simulink model "ME19B031_PROJECT_2"  (R2021a)
settings: Solver=VariableStepAuto  StartTime=0.0  StopTime=10.0  RelTol=1e-3
libraries: simulink_extras x7, pid_lib x2
settings Model: Creator=nayin  LastModifiedBy=nayin
settings SolverCC: ZeroCrossAlgorithm=Adaptive
settings DebuggingCC: IgnoredZcDiagnostic=none

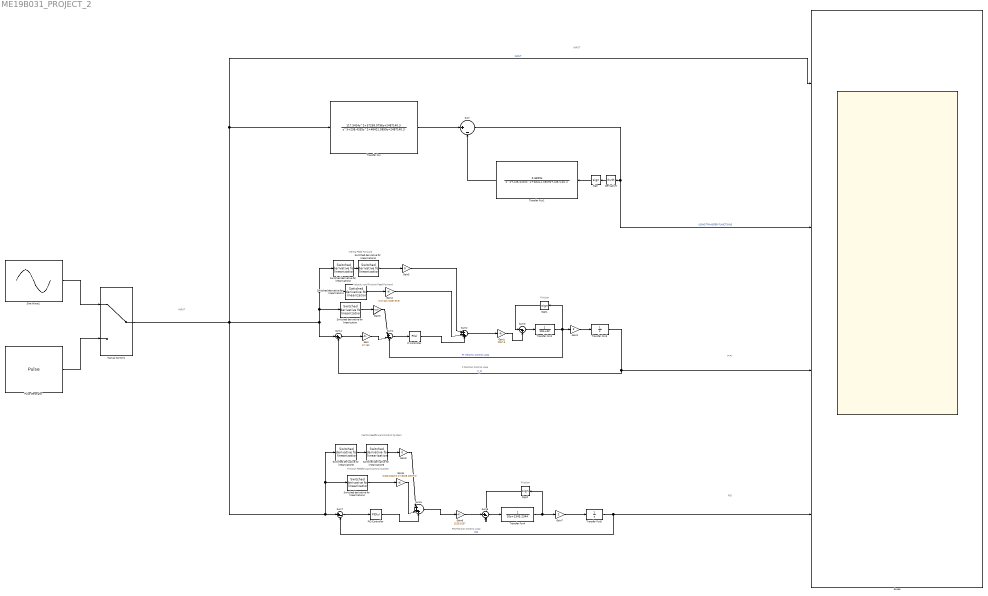
== system ME19B031_PROJECT_2 ==
  note: INPUT
  note: INPUT
  note: PID
  note: P-PI
  note: Velocity and Friction Feed Forward
  note: Inertia Feed Forward
  note: Friction
  note: P Position Control Loop
  note: PID Position Control Loop
  note: Inertia Feedforward Control System
  note: Friction Feedforward Control System
  note: Friction
  Derivative : Derivative
  Gain : Gain  Gain=37.133
  Gain1 : Gain  Gain=2057.6
  Gain2 : Gain  Gain=3
  Gain3 : Gain  Gain=0.5/3
  Gain4 : Gain  Gain=(0.1*42)/(2057.6*3)
  Gain5 : Gain  Gain=0
  Gain6 : Gain  Gain=3228.1057
  Gain7 : Gain  Gain=3
  Gain8 : Gain  Gain=(1343.2344*0.1)/(3228.1057*3)
  Gain9 : Gain  Gain=0
  Manual Switch1 : ManualSwitch
  PI Controller : pid_lib/PID Controller  Controller=PI  Form=Parallel  TimeDomain=Continuous-time  UseExternalTs=off  SampleTime=-1  IntegratorMethod=Forward Euler  FilterMethod=Forward Euler  ControllerParametersSource=internal  P=1.13838  I=108.5  D=0  UseFilter=on  N=100  TunerSelectOption=Transfer Function Based (PID Tuner App)  InitialConditionSource=internal  InitialConditionForIntegrator=0  InitialConditionForFilter=0  DifferentiatorICPrevScaledInput=0  ExternalReset=none  TrackingMode=off  Kt=1  LimitOutput=off  SatLimitsSource=internal  UpperSaturationLimit=inf  LowerSaturationLimit=-inf  LinearizeAsGain=on  AntiWindupMode=none  Kb=1  POutMin=[]  POutMax=[]  IOutMin=[]  IOutMax=[]  DOutMin=[]  DOutMax=[]  NOutMin=[]  NOutMax=[]  SumOutMin=[]  SumOutMax=[]  SaturationOutMin=[]  SaturationOutMax=[]  PParamMin=[]  PParamMax=[]  IParamMin=[]  IParamMax=[]  DParamMin=[]  DParamMax=[]  NParamMin=[]  NParamMax=[]  KbParamMin=[]  KbParamMax=[]  KtParamMin=[]  KtParamMax=[]  KbOutMin=[]  KbOutMax=[]  KtOutMin=[]  KtOutMax=[]  IntegratorOutMin=[]  IntegratorOutMax=[]  FilterOutMin=[]  FilterOutMax=[]  SumI1OutMin=[]  SumI1OutMax=[]  SumI2OutMin=[]  SumI2OutMax=[]  SumI3OutMin=[]  SumI3OutMax=[]  SumI4OutMin=[]  SumI4OutMax=[]  SumDOutMin=[]  SumDOutMax=[]  DifferentiatorOutMin=[]  DifferentiatorOutMax=[]  FilterDiffOutCoefMin=[]  FilterDiffOutCoefMax=[]  ReciprocalOutMin=[]  ReciprocalOutMax=[]  SumDenOutMin=[]  SumDenOutMax=[]  SumNumOutMin=[]  SumNumOutMax=[]  DivideOutMin=[]  DivideOutMax=[]  UdiffTsProdOutMin=[]  UdiffTsProdOutMax=[]  NTsProdOutMin=[]  NTsProdOutMax=[]  UintegralTsProdOutMin=[]  UintegralTsProdOutMax=[]  UngainTsProdOutMin=[]  UngainTsProdOutMax=[]  IntegratorContinuousStateAttributes=''  IntegratorStateMustResolveToSignalObject=off  IntegratorRTWStateStorageClass=Auto  FilterContinuousStateAttributes=''  FilterStateMustResolveToSignalObject=off  FilterRTWStateStorageClass=Auto  ParallelPVariant=InternalParameters  IdealPVariant=Disabled  IVariant=InternalParameters  DVariant=Disabled  IntegratorVariant=Continuous  SatVariant=Disabled  AWVariant=Passthrough  PCopyVariant=Disabled  TRVariant=Disabled  FdbkBlocksVariant=Forward  IdealPFdbkVariant=Disabled  SatFdbkVariant=Disabled  DerivativeFilterVariant=Disabled  NVariant=Disabled  NCopyVariant=Disabled_SignalSpec  FilterICVariant=Disabled  IntegratorICVariant=InternalICs  ExternalResetVariant=Disabled  TRSumVariant=Passthrough  SumFdbkVariant=Disabled  SumVariant=Sum_PI  TsampFilterVariant=InternalTs  TsampNgainVariant=Passthrough  TsampIntegralVariant=Passthrough  ExternalSaturationOutDataTypeStr=Inherit: Same as second input
  PID Controller : pid_lib/PID Controller  Controller=PID  Form=Parallel  TimeDomain=Continuous-time  UseExternalTs=off  SampleTime=-1  IntegratorMethod=Forward Euler  FilterMethod=Forward Euler  ControllerParametersSource=internal  P=50  I=2568.2141  D=2.323356  UseFilter=on  N=100  TunerSelectOption=Transfer Function Based (PID Tuner App)  InitialConditionSource=internal  InitialConditionForIntegrator=0  InitialConditionForFilter=0  DifferentiatorICPrevScaledInput=0  ExternalReset=none  TrackingMode=off  Kt=1  LimitOutput=off  SatLimitsSource=internal  UpperSaturationLimit=inf  LowerSaturationLimit=-inf  LinearizeAsGain=on  AntiWindupMode=none  Kb=1  POutMin=[]  POutMax=[]  IOutMin=[]  IOutMax=[]  DOutMin=[]  DOutMax=[]  NOutMin=[]  NOutMax=[]  SumOutMin=[]  SumOutMax=[]  SaturationOutMin=[]  SaturationOutMax=[]  PParamMin=[]  PParamMax=[]  IParamMin=[]  IParamMax=[]  DParamMin=[]  DParamMax=[]  NParamMin=[]  NParamMax=[]  KbParamMin=[]  KbParamMax=[]  KtParamMin=[]  KtParamMax=[]  KbOutMin=[]  KbOutMax=[]  KtOutMin=[]  KtOutMax=[]  IntegratorOutMin=[]  IntegratorOutMax=[]  FilterOutMin=[]  FilterOutMax=[]  SumI1OutMin=[]  SumI1OutMax=[]  SumI2OutMin=[]  SumI2OutMax=[]  SumI3OutMin=[]  SumI3OutMax=[]  SumI4OutMin=[]  SumI4OutMax=[]  SumDOutMin=[]  SumDOutMax=[]  DifferentiatorOutMin=[]  DifferentiatorOutMax=[]  FilterDiffOutCoefMin=[]  FilterDiffOutCoefMax=[]  ReciprocalOutMin=[]  ReciprocalOutMax=[]  SumDenOutMin=[]  SumDenOutMax=[]  SumNumOutMin=[]  SumNumOutMax=[]  DivideOutMin=[]  DivideOutMax=[]  UdiffTsProdOutMin=[]  UdiffTsProdOutMax=[]  NTsProdOutMin=[]  NTsProdOutMax=[]  UintegralTsProdOutMin=[]  UintegralTsProdOutMax=[]  UngainTsProdOutMin=[]  UngainTsProdOutMax=[]  IntegratorContinuousStateAttributes=''  IntegratorStateMustResolveToSignalObject=off  IntegratorRTWStateStorageClass=Auto  FilterContinuousStateAttributes=''  FilterStateMustResolveToSignalObject=off  FilterRTWStateStorageClass=Auto  ParallelPVariant=InternalParameters  IdealPVariant=Disabled  IVariant=InternalParameters  DVariant=InternalParameters  IntegratorVariant=Continuous  SatVariant=Disabled  AWVariant=Passthrough  PCopyVariant=Disabled  TRVariant=Disabled  FdbkBlocksVariant=Forward  IdealPFdbkVariant=Disabled  SatFdbkVariant=Disabled  DerivativeFilterVariant=ContFilter  NVariant=InternalParameters  NCopyVariant=Disabled  FilterICVariant=InternalICsFilter  IntegratorICVariant=InternalICs  ExternalResetVariant=Disabled  TRSumVariant=Passthrough  SumFdbkVariant=Disabled  SumVariant=Sum_PID  TsampFilterVariant=InternalTs  TsampNgainVariant=Passthrough  TsampIntegralVariant=Passthrough  ExternalSaturationOutDataTypeStr=Inherit: Same as second input
  Pulse Generator : DiscretePulseGenerator  PulseType=Time based  Period=1  PulseWidth=50
  Scope : Scope  NumInputPorts=4
  Sign : Signum  ZeroCross=off
  Sign1 : Signum
  Sign2 : Signum
  Sine Wave1 : Sin  SampleTime=0
  Sum{,4,6..7} (4 alike) : Sum  Inputs=|+-
  Sum1 : Sum  Inputs=|++-
  Sum2 : Sum  Inputs=|+++
  Sum3 : Sum  Inputs=|-+
  Sum5 : Sum  Inputs=|+++
  Switched derivative for linearization{,1..6} (7 alike) : simulink_extras/Linearization/Switched derivative for linearization  switchVal=0  derivConst=100
      settings: SourceProductBaseCode=SL
  Transfer Fcn : TransferFcn  Numerator=[117.5424 37258.9796 2487140.3]  Denominator=[ 1 238.4335 48421.5859 2487140.3]
  Transfer Fcn1 : TransferFcn  Numerator=[2.6815 0]  Denominator=[ 1 238.4335 48421.5859 2487140.3]
  Transfer Fcn2 : TransferFcn  Denominator=[10 42]
  Transfer Fcn3 : TransferFcn  Denominator=[1 0]
  Transfer Fcn4 : TransferFcn  Denominator=[10 1343.2344]
  Transfer Fcn5 : TransferFcn  Denominator=[1 0]
  wires:
  Pulse Generator/1 -> Manual Switch1/2
  Sine Wave1/1 -> Manual Switch1/1
  Sign/1 -> Transfer Fcn1/1
  Derivative/1 -> Sign/1
  Transfer Fcn1/1 -> Sum/2
  Sum/1 -> Derivative/1, Scope/2  "USING TRANSFER FUNCTIONS"
  Transfer Fcn/1 -> Sum/1
  Gain5/1 -> Sum2/1
  Sum2/1 -> Gain1/1
  Switched derivative for linearization1/1 -> Gain4/1
  Gain4/1 -> Sum2/2
  PI Controller/1 -> Sum2/3
  Switched derivative for linearization2/1 -> Switched derivative for linearization3/1
  Switched derivative for linearization3/1 -> Gain5/1
  Sum3/1 -> Transfer Fcn2/1
  Transfer Fcn3/1 -> Sum4/2, Scope/3  "P_PI"
  Gain1/1 -> Sum3/2
  Sum4/1 -> Gain/1
  Gain3/1 -> Sum1/1
  Sum1/1 -> PI Controller/1
  Switched derivative for linearization/1 -> Gain3/1
  Gain2/1 -> Transfer Fcn3/1
  Sign1/1 -> Sum3/1
  Transfer Fcn2/1 -> Sum1/3, Sign1/1, Gain2/1  "PI Velocity Control Loop"
  Gain/1 -> Sum1/2
  PID Controller/1 -> Sum5/3
  Gain7/1 -> Transfer Fcn5/1
  Transfer Fcn5/1 -> Scope/4, Sum7/2  "PID"
  Transfer Fcn4/1 -> Sign2/1, Gain7/1
  Gain9/1 -> Sum5/1
  Sum7/1 -> PID Controller/1
  Sign2/1 -> Sum6/2
  Manual Switch1/1 -> Switched derivative for linearization4/1, Switched derivative for linearization5/1, Sum7/1, Sum4/1, Switched derivative for linearization/1, Switched derivative for linearization2/1, Switched derivative for linearization1/1, Transfer Fcn/1, Scope/1  "INPUT"
  Sum5/1 -> Gain6/1
  Switched derivative for linearization4/1 -> Gain8/1
  Switched derivative for linearization6/1 -> Gain9/1
  Gain6/1 -> Sum6/1
  Sum6/1 -> Transfer Fcn4/1
  Gain8/1 -> Sum5/2
  Switched derivative for linearization5/1 -> Switched derivative for linearization6/1
